simulink model "MODEL"  (R2023a)
settings: Solver=VariableStepAuto  StartTime=0.0  StopTime=10  RelTol=1e-2
values from neighbouring files (symbols this model uses):
  A = [0 1 0 0 0 ... (first row only)    [Main.m]    (also in SweepTest.m; myActiveSuspensions.mat = [0 -861.462979483 0 763.157894737 0 1 -89.1168599465 0 78.94)
  A_lift = 3    [Main.m]    (also in SweepTest.m; myActiveSuspensions.mat)
  B1 = [0;0;0;0;mi*gamma]    [Main.m]    (also in SweepTest.m; myActiveSuspensions.mat = [0 0 0 0 154.5])
  B2 = [0 0 0 0 0 0 ... (first row only)    [Main.m]    (also in SweepTest.m; myActiveSuspensions.mat = [0 0 0 -1 0 0 0.00338983050847 0 0 0 0 0 ... (30 elements, 5)
  C = [1 0 0 0 0 ... (first row only)    [Main.m]    (also in SweepTest.m; myActiveSuspensions.mat = [1 1 -98.3050847458 0 0 -10.1694915254 0 1 0 0 0 0 ... (15 e)
  Cd_lift = 0.5    [Main.m]    (also in SweepTest.m; myActiveSuspensions.mat)
  Ce = [1 0 0 0 0]    [Main.m]    (also in SweepTest.m; myActiveSuspensions.mat)
  D1 = [0;0;0]    [Main.m]    (also in SweepTest.m; myActiveSuspensions.mat = [0 0 0])
  D2 = [0 0 1 0 0 0 ... (first row only)    [Main.m]    (also in SweepTest.m; myActiveSuspensions.mat = [0 0 0 0 0 0.00338983050847 1 0 0 0 1 0 ... (18 elements, 3x)
  De1 = 0    [Main.m]    (also in SweepTest.m; myActiveSuspensions.mat)
  De2 = [0 0 1 0 0 -1]    [Main.m]    (also in SweepTest.m; myActiveSuspensions.mat)
  DT = 1e-4    (= 0.0001)    [Main.m]    (also in SweepTest.m; myActiveSuspensions.mat)
  n = size(V)    [JCF.m]    (also in Main.m = 5; SweepTest.m = 5; myActiveSuspensions.mat = 5)
  p = 1    [Main.m]    (also in SweepTest.m; myActiveSuspensions.mat)
  r = nd + q + m    (= 6)    [Main.m]    (also in SweepTest.m; myActiveSuspensions.mat)
  r0 = - g*ms/ks + l0s + Lift/ks    (= 0.597040517241)    [Main.m]    (also in SweepTest.m; myActiveSuspensions.mat)
  rho_lift = 1.225    [Main.m]    (also in SweepTest.m; myActiveSuspensions.mat)
  v = 10    [Main.m]    (also in SweepTest.m; myActiveSuspensions.mat)
  w0 = [d0; nu0; r0]    [Main.m]    (also in SweepTest.m; myActiveSuspensions.mat = [0 -91.875 0 0 0 0.597040517241])
  x_init = [(- g*ms/ks + l0s + Lift/ks) - Diseq ... (first row only)    [Main.m]    (also in SweepTest.m; myActiveSuspensions.mat = [0.597040517241 0 0.3385371843 0 0])
  x_tilde_init = x_init - x0    [Main.m]    (also in SweepTest.m; myActiveSuspensions.mat = [0 0 0 0 0])
libraries: simulink x3
settings Model: Creator=aleze  LastModifiedBy=aleze

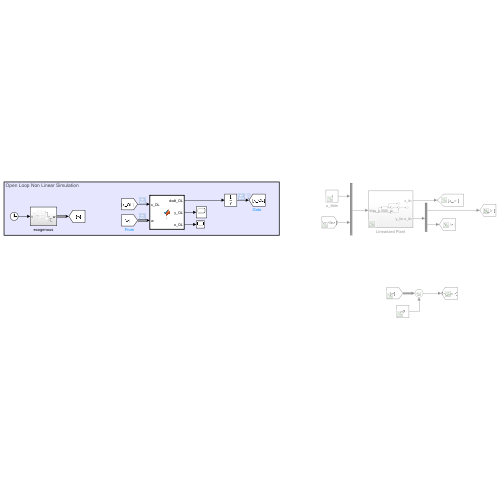
[thumbnail: Simulink's stored preview of the top-level diagram]
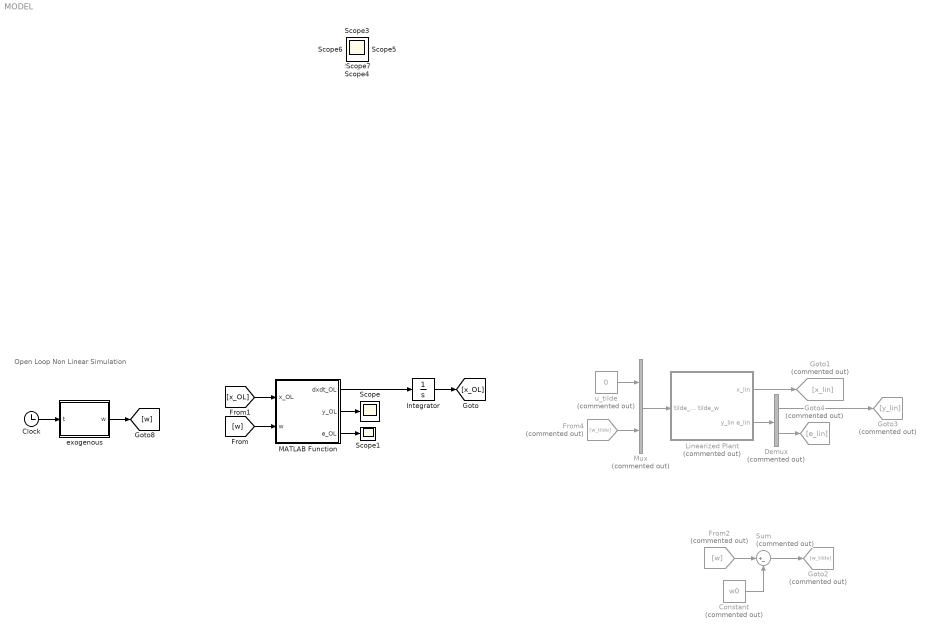
== system MODEL ==
  note: Open Loop Non Linear Simulation
  Clock : Clock
  Constant : Constant  Commented=on  Value=w0
  Demux : Demux  Commented=on  Outputs=2
  From2 : From  Commented=on  GotoTag=w
  From4 : From  Commented=on  GotoTag=w_tilde
  Goto1 : Goto  Commented=on  GotoTag=x_lin
  Goto2 : Goto  Commented=on  GotoTag=w_tilde
  Goto3 : Goto  Commented=on  GotoTag=y_lin
  Goto4 : Goto  Commented=on  GotoTag=e_lin
  Integrator : Integrator  InitialCondition=x_init
  Linearized Plant : Subsystem  Commented=on
  MATLAB Function : MATLAB Function  TreatAsAtomicUnit=on
  Mux : Mux  Commented=on  Inputs=2
  Scope{,1..7} (8 alike) : Scope
  Sum : Sum  Commented=on  Inputs=|+-
  exogenous : Subsystem
  u_tilde : Constant  Commented=on  Value=0
  wires:
  Clock/1 -> exogenous/1(t)
  exogenous/1(w) -> [w]
  [w] -> MATLAB Function/2(w)
  MATLAB Function/1(dxdt_OL) -> Integrator/1
  MATLAB Function/3(e_OL) -> Scope1/1
  Integrator/1 -> [x_OL]
  [x_OL] -> MATLAB Function/1(x_OL)
  From2/1 -> Sum/1
  Constant/1 -> Sum/2
  Sum/1 -> Goto2/1
  From4/1 -> Mux/2
  Mux/1 -> Linearized Plant/1(tilde_u tilde_w)
  Linearized Plant/2(y_lin e_lin) -> Demux/1
  Demux/1 -> Goto3/1
  Demux/2 -> Goto4/1
  Linearized Plant/1(x_lin) -> Goto1/1
  MATLAB Function/2(y_OL) -> Scope/1
  u_tilde/1 -> Mux/1

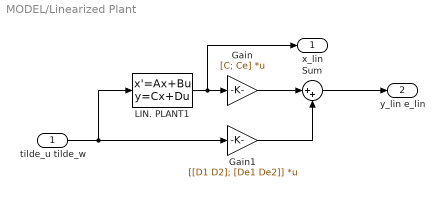
== system MODEL/Linearized Plant ==
  tilde_u tilde_w : Inport
  Gain : Gain  Gain=[C; Ce]  Multiplication=Matrix(K*u)
  Gain1 : Gain  Gain=[[D1 D2]; [De1 De2]]  Multiplication=Matrix(K*u)
  LIN. PLANT1 : StateSpace  A=A  B=[B1 B2]  C=eye(n)  D=zeros(n,p+r)  InitialCondition=x_tilde_init
  Sum : Sum  Inputs=|++
  x_lin : Outport
  y_lin e_lin : Outport  Port=2
  wires:
  LIN. PLANT1/1 -> x_lin/1, Gain/1
  tilde_u tilde_w/1 -> LIN. PLANT1/1, Gain1/1
  Gain1/1 -> Sum/2
  Gain/1 -> Sum/1
  Sum/1 -> y_lin e_lin/1

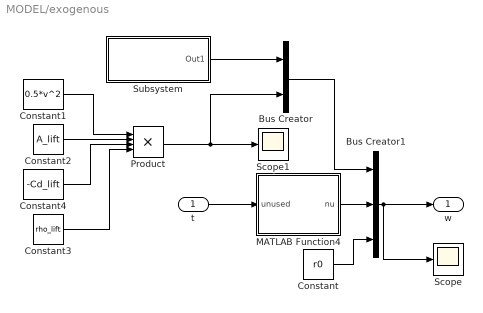
== system MODEL/exogenous ==
  t : Inport
  Bus Creator : BusCreator  Inputs=2
  Bus Creator1 : BusCreator  Inputs=3
  Constant : Constant  Value=r0
  Constant1 : Constant  Value=0.5*v^2  SampleTime=DT
  Constant2 : Constant  Value=A_lift  SampleTime=DT
  Constant3 : Constant  Value=rho_lift  SampleTime=DT
  Constant4 : Constant  Value=-Cd_lift  SampleTime=DT
  MATLAB Function4 : MATLAB Function  TreatAsAtomicUnit=on  SystemSampleTime=DT
  Product : Product  Inputs=4
  Scope : Scope
  Scope1 : Scope
  Subsystem : Subsystem
  w : Outport
  wires:
  Constant1/1 -> Product/1
  Subsystem/1(Out1) -> Bus Creator/1
  Constant2/1 -> Product/2
  t/1 -> MATLAB Function4/1(unused)
  Constant3/1 -> Product/4
  Constant4/1 -> Product/3
  Product/1 -> Bus Creator/2, Scope1/1
  Bus Creator/1 -> Bus Creator1/1
  MATLAB Function4/1(nu) -> Bus Creator1/2
  Constant/1 -> Bus Creator1/3
  Bus Creator1/1 -> Scope/1, w/1

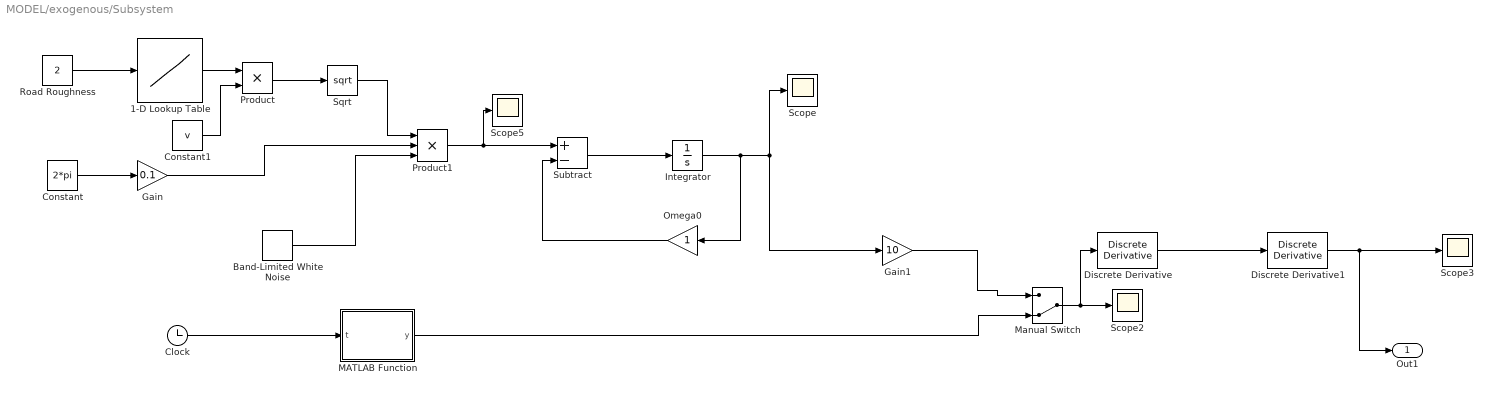
== system MODEL/exogenous/Subsystem ==
  1-D Lookup Table : Lookup_n-D  NumberOfTableDimensions=1  BreakpointsForDimension1=[1;2;3;4;5;6;7;8]  Table=[1.6e-05;6.4e-05;0.000256;0.001024;0.004096;0.016384;0.065536;0.262144]  InternalRulePriority=Speed  RndMeth=Simplest
  Band-Limited White Noise : simulink/Sources/Band-Limited White Noise  Cov=0.1  Ts=0.01  seed=[23341]
  Clock : Clock
  Constant : Constant  Value=2*pi
  Constant1 : Constant  Value=v
  Discrete Derivative : simulink/Quick Insert/Discrete/Discrete Derivative  gainval=1.0  ICPrevScaledInput=0.0  OutMin=[]  OutMax=[]  OutDataType=fixdt(1, 16)  OutScaling=2^-10  DoSatur=off
  Discrete Derivative1 : simulink/Quick Insert/Discrete/Discrete Derivative  gainval=1.0  ICPrevScaledInput=0.0  OutMin=[]  OutMax=[]  OutDataType=fixdt(1, 16)  OutScaling=2^-10  DoSatur=off
  Gain : Gain  Gain=0.1
  Gain1 : Gain  Gain=10
  Integrator : Integrator
  MATLAB Function : MATLAB Function  TreatAsAtomicUnit=on
  Manual Switch : ManualSwitch  CurrentSetting=0
  Omega0 : Gain
  Product : Product
  Product1 : Product  Inputs=3
  Road Roughness : Constant  Value=2
  Scope{,2..3,5} (4 alike) : Scope
  Sqrt : Sqrt
  Subtract : Sum  Inputs=+-
  Out1 : Outport
  wires:
  Subtract/1 -> Integrator/1
  Road Roughness/1 -> 1-D Lookup Table/1
  Clock/1 -> MATLAB Function/1(t)
  1-D Lookup Table/1 -> Product/1
  Sqrt/1 -> Product1/1
  Constant/1 -> Gain/1
  Band-Limited White Noise/1 -> Product1/3
  Omega0/1 -> Subtract/2
  MATLAB Function/1(y) -> Manual Switch/2
  Product1/1 -> Scope5/1, Subtract/1
  Integrator/1 -> Omega0/1, Gain1/1, Scope/1
  Constant1/1 -> Product/2
  Product/1 -> Sqrt/1
  Gain/1 -> Product1/2
  ? -> ?
  Gain1/1 -> Manual Switch/1
  Discrete Derivative/1 -> Discrete Derivative1/1
  Discrete Derivative1/1 -> Out1/1, Scope3/1
  Manual Switch/1 -> Scope2/1, Discrete Derivative/1

== matlab function MODEL/MATLAB Function ==
  data: dxdt_OL output; x_OL input; y_OL output; w input; e_OL output
function [dxdt_OL, y_OL, e_OL] = f(x_OL,w)

x1 = x_OL(1);
x2 = x_OL(2);
x3 = x_OL(3);
x4 = x_OL(4);

% Disturbance
d=w(1);
Lift = w(2);

% Noise
ni1 = w(3);
ni2 = w(4);
ni3 = w(5);

% Reference
r0 = w(6);

mi = 1e-7; % scale coefficient to improve numerical conditioning of P
Ap = 3.35e-4; % m^2
%% ACTUAL PLANT PARAMETERS

%% Plant Parameters
ks = 29300; %spring coefficient
mu = 38;
ms = 395;
l0s = 0.5;
g = 9.81;
betas = 3000; %damping coefficient 
mi = 1e-7; % scale coefficient to improve numerical conditioning of P

barm = (mu+ms)/ms; 

%% STATE DYNAMICS
dxdt_OL = [x2
    barm/mu*(-ks*(x1-l0s)-betas*x2)-1/mu*ft(x3)+ Lift/ms
    x4
    -g+ks/mu*(x1-l0s)+betas/mu*x2+1/mu*ft(x3)-d
    0];

%% Model equations 
% dxdt = [x(2) 
%     -M*ks*(x(1)-l0s)-M*betas*x(2)-(1/mu)*ft(x(3)) %+M*(Ap/mi)*x(5) +Lift/ms       %+kt/mu*(x(3)-l0t)
%     x(4) 
%     -g+(1/mu)*ft(x(3))+(ks/mu)*(x(1)-l0s)+(betas/mu)*x(2)-d1  %-1/mu*Ap/mi*x(5)      %-kt/mu*(x(3)-l0t)
%     -beta*x(5)-mi*alfa*Ap*x(2)]; 
 
y_OL = [x_OL(1)+ni1 
     x_OL(1)+x_OL(3)+ni2 
     1/ms*(Lift-ms*g-ks*(x_OL(1)-l0s)-betas*x_OL(2)+x_OL(5)*Ap/mi)+ni3];

e_OL = x_OL(1) + ni1 -r0;
end


%% SUPPORT FUNCTIONS

function f = ft(s)
l0t = 0.10; 
kt = 290000; %tyre elastic coefficient
if s > l0t
    f = 0;
else
    f = -kt*(s-l0t);
end
end

== matlab function MODEL/exogenous/Subsystem/MATLAB Function ==
  data: t input; y output
function y = fcn(t)
k = 10; % parametro dipendente da v
d = 2;%s, displacement 
if t<(d - (0.6/k))
    y=0;
    
else
    if t>(d + (0.6/k))
        y=0;
    else
   y = ((15)/(16))*((0.045)/(0.6))*(((k*(t-d))/(0.6))^(4)-2*((k*(t-d))/(0.6))^(2)+1);
    end
end

== matlab function MODEL/exogenous/MATLAB Function4 ==
  data: unused input; nu output
function nu = noises(~)
std_pot = 0.001; % [m] potentiomenter standard deviation
std_laser = 0.001; %standard deviation laser
std_acc = 110e-6*sqrt(200); % [m/s^2] accelerometer standard deviation
nu = [std_pot*(2*rand(1)-1)
      std_laser*(2*rand(1)-1)
      std_acc*(2*rand(1)-1)];

end
